simulink model "FOC_PI_5phase"  (R2024b)
settings: Solver=VariableStepAuto  StartTime=0.0  StopTime=0.5  RelTol=1e-3
InitFcn:
  | Pn=4;
  | Ld=1.35e-3;
  | Lq=1.35e-3;
  | R=2.875;
  | flux=0.05;
  | J=0.002;
  | B=0.02;
  | fc=470;
libraries: spsIGBTDiodeLib x10, slpidlib x3, simulink x1, spsDCVoltageSourceLib x1, spsPermanentMagnetSynchronousMachineLib x1, spsVoltageMeasurementLib x1, sps_lib x1
settings Model: Creator=23954  LastModifiedBy=23954

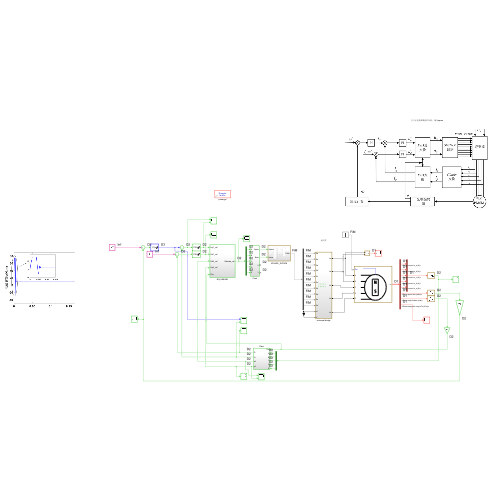
[thumbnail: Simulink's stored preview of the top-level diagram]
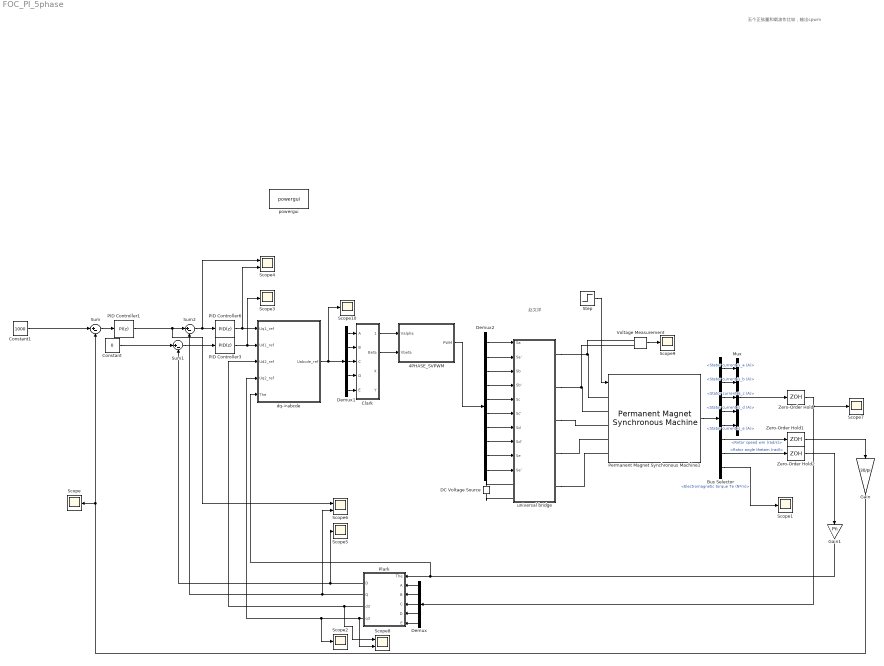
== system FOC_PI_5phase ==
  note: 赵文祥
  note: 五个正弦量和载波作比较，输出spwm
  4PHASE_SVPWM : Subsystem
  Bus Selector : BusSelector  OutputSignals=Stator current is_a (A),Stator current is_b (A),Stator current is_c (A),Stator current is_d (A),Stator current is_e (A),Rotor speed wm (rad/s),Rotor angle thetam (rad),Electromagnetic torque Te (N*m)
  Clark : Subsystem
  Constant : Constant  Value=0
  Constant1 : Constant  Value=1000
  DC Voltage Source : spsDCVoltageSourceLib/DC Voltage Source  Amplitude=311  Measurements=None
  Demux : Demux  Outputs=5
  Demux1 : Demux  Outputs=5
  Demux2 : Demux  Outputs=10
  Gain : Gain  Gain=30/pi
  Gain1 : Gain  Gain=Pn
  Mux : Mux  Inputs=5
  PID Controller1 : slpidlib/PID Controller  Controller=PI  Form=Parallel  TimeDomain=Discrete-time  UseExternalTs=off  SampleTime=1e-3  IntegratorMethod=Forward Euler  FilterMethod=Forward Euler  ControllerParametersSource=internal  P=5*J/1.5/Pn/flux  I=10*10*J/1.5/Pn/flux  UseKiTs=off  D=0  UseExternalDerivativeSource=off  N=100  UseFilter=on  TunerSelectOption=Transfer Function Based (PID Tuner App)  InitialConditionSource=internal  InitialConditionForIntegrator=0  InitialConditionForFilter=0  DifferentiatorICPrevScaledInput=0  ExternalReset=none  TrackingMode=off  Kt=1  LimitOutput=on  SatLimitsSource=internal  UpperSaturationLimit=150  LowerSaturationLimit=-150  LinearizeAsGain=on  AntiWindupMode=none  Kb=1  LimitIntegrator=off  UpperIntegratorSaturationLimit=inf  LowerIntegratorSaturationLimit=-inf  POutMin=[]  POutMax=[]  IOutMin=[]  IOutMax=[]  DOutMin=[]  DOutMax=[]  NOutMin=[]  NOutMax=[]  SumOutMin=[]  SumOutMax=[]  SaturationOutMin=[]  SaturationOutMax=[]  PParamMin=[]  PParamMax=[]  IParamMin=[]  IParamMax=[]  DParamMin=[]  DParamMax=[]  NParamMin=[]  NParamMax=[]  KbParamMin=[]  KbParamMax=[]  KtParamMin=[]  KtParamMax=[]  KbOutMin=[]  KbOutMax=[]  KtOutMin=[]  KtOutMax=[]  IntegratorOutMin=[]  IntegratorOutMax=[]  FilterOutMin=[]  FilterOutMax=[]  SumI1OutMin=[]  SumI1OutMax=[]  SumI2OutMin=[]  SumI2OutMax=[]  SumI3OutMin=[]  SumI3OutMax=[]  SumI4OutMin=[]  SumI4OutMax=[]  SumDOutMin=[]  SumDOutMax=[]  DifferentiatorOutMin=[]  DifferentiatorOutMax=[]  FilterDiffOutCoefMin=[]  FilterDiffOutCoefMax=[]  ReciprocalOutMin=[]  ReciprocalOutMax=[]  SumDenOutMin=[]  SumDenOutMax=[]  SumNumOutMin=[]  SumNumOutMax=[]  DivideOutMin=[]  DivideOutMax=[]  UdiffTsProdOutMin=[]  UdiffTsProdOutMax=[]  NTsProdOutMin=[]  NTsProdOutMax=[]  UintegralTsProdOutMin=[]  UintegralTsProdOutMax=[]  UngainTsProdOutMin=[]  UngainTsProdOutMax=[]  ClampingZeroOutDataTypeStr=Inherit: Inherit via back propagation  ClampingZeroOutMin=[]  ClampingZeroOutMax=[]  FilterDenConstantOutDataTypeStr=Inherit: Inherit via back propagation  FilterDenConstantOutMin=[]  FilterDenConstantOutMax=[]  PCopyOutDataTypeStr=Inherit: Inherit via back propagation  PCopyOutMin=[]  PCopyOutMax=[]  NCopyOutDataTypeStr=Inherit: Inherit via back propagation  NCopyOutMin=[]  NCopyOutMax=[]  IntegratorContinuousStateAttributes=''  IntegratorStateMustResolveToSignalObject=off  IntegratorRTWStateStorageClass=Auto  FilterContinuousStateAttributes=''  FilterStateMustResolveToSignalObject=off  FilterRTWStateStorageClass=Auto  ParallelPVariant=InternalParameters  IdealPVariant=Disabled  IVariant=InternalParameters  DVariant=Disabled  IntegratorVariant=Discrete  SatVariant=Enabled  AWVariant=Passthrough  PCopyVariant=Disabled  TRVariant=Disabled  FdbkBlocksVariant=Forward  IdealPFdbkVariant=Disabled  SatFdbkVariant=Disabled  DerivativeFilterVariant=Disabled  NVariant=Disabled  NCopyVariant=Disabled_SignalSpec  FilterICVariant=Disabled  IntegratorICVariant=InternalICs  ExternalResetVariant=Disabled  TRSumVariant=Passthrough  SumFdbkVariant=Disabled  SumVariant=Sum_PI  TsampFilterVariant=InternalTs  TsampNgainVariant=Passthrough  TsampIntegralVariant=Disabled_SignalSpec  ExternalSaturationOutDataTypeStr=Inherit: Same as second input  DerivativeSourceVariant=Disabled  PreIntVariant=InternalPreInt
  PID Controller3 : slpidlib/PID Controller  Controller=PID  Form=Parallel  TimeDomain=Discrete-time  UseExternalTs=off  SampleTime=1e-4  IntegratorMethod=Forward Euler  FilterMethod=Forward Euler  ControllerParametersSource=internal  P=2*pi*fc*Ld  I=2*pi*fc*R  UseKiTs=off  D=0  UseExternalDerivativeSource=off  N=100  UseFilter=on  TunerSelectOption=Transfer Function Based (PID Tuner App)  InitialConditionSource=internal  InitialConditionForIntegrator=0  InitialConditionForFilter=0  DifferentiatorICPrevScaledInput=0  ExternalReset=none  TrackingMode=off  Kt=1  LimitOutput=on  SatLimitsSource=internal  UpperSaturationLimit=150  LowerSaturationLimit=-150  LinearizeAsGain=on  AntiWindupMode=none  Kb=1  LimitIntegrator=off  UpperIntegratorSaturationLimit=inf  LowerIntegratorSaturationLimit=-inf  POutMin=[]  POutMax=[]  IOutMin=[]  IOutMax=[]  DOutMin=[]  DOutMax=[]  NOutMin=[]  NOutMax=[]  SumOutMin=[]  SumOutMax=[]  SaturationOutMin=[]  SaturationOutMax=[]  PParamMin=[]  PParamMax=[]  IParamMin=[]  IParamMax=[]  DParamMin=[]  DParamMax=[]  NParamMin=[]  NParamMax=[]  KbParamMin=[]  KbParamMax=[]  KtParamMin=[]  KtParamMax=[]  KbOutMin=[]  KbOutMax=[]  KtOutMin=[]  KtOutMax=[]  IntegratorOutMin=[]  IntegratorOutMax=[]  FilterOutMin=[]  FilterOutMax=[]  SumI1OutMin=[]  SumI1OutMax=[]  SumI2OutMin=[]  SumI2OutMax=[]  SumI3OutMin=[]  SumI3OutMax=[]  SumI4OutMin=[]  SumI4OutMax=[]  SumDOutMin=[]  SumDOutMax=[]  DifferentiatorOutMin=[]  DifferentiatorOutMax=[]  FilterDiffOutCoefMin=[]  FilterDiffOutCoefMax=[]  ReciprocalOutMin=[]  ReciprocalOutMax=[]  SumDenOutMin=[]  SumDenOutMax=[]  SumNumOutMin=[]  SumNumOutMax=[]  DivideOutMin=[]  DivideOutMax=[]  UdiffTsProdOutMin=[]  UdiffTsProdOutMax=[]  NTsProdOutMin=[]  NTsProdOutMax=[]  UintegralTsProdOutMin=[]  UintegralTsProdOutMax=[]  UngainTsProdOutMin=[]  UngainTsProdOutMax=[]  ClampingZeroOutDataTypeStr=Inherit: Inherit via back propagation  ClampingZeroOutMin=[]  ClampingZeroOutMax=[]  FilterDenConstantOutDataTypeStr=Inherit: Inherit via back propagation  FilterDenConstantOutMin=[]  FilterDenConstantOutMax=[]  PCopyOutDataTypeStr=Inherit: Inherit via back propagation  PCopyOutMin=[]  PCopyOutMax=[]  NCopyOutDataTypeStr=Inherit: Inherit via back propagation  NCopyOutMin=[]  NCopyOutMax=[]  IntegratorContinuousStateAttributes=''  IntegratorStateMustResolveToSignalObject=off  IntegratorRTWStateStorageClass=Auto  FilterContinuousStateAttributes=''  FilterStateMustResolveToSignalObject=off  FilterRTWStateStorageClass=Auto  ParallelPVariant=InternalParameters  IdealPVariant=Disabled  IVariant=InternalParameters  DVariant=InternalParameters  IntegratorVariant=Discrete  SatVariant=Enabled  AWVariant=Passthrough  PCopyVariant=Disabled  TRVariant=Disabled  FdbkBlocksVariant=Forward  IdealPFdbkVariant=Disabled  SatFdbkVariant=Disabled  DerivativeFilterVariant=ForwardEulerFilter  NVariant=InternalParameters  NCopyVariant=Disabled  FilterICVariant=InternalICsFilter  IntegratorICVariant=InternalICs  ExternalResetVariant=Disabled  TRSumVariant=Passthrough  SumFdbkVariant=Disabled  SumVariant=Sum_PID  TsampFilterVariant=InternalTs  TsampNgainVariant=Passthrough  TsampIntegralVariant=Disabled_SignalSpec  ExternalSaturationOutDataTypeStr=Inherit: Same as second input  DerivativeSourceVariant=ErrorSignal  PreIntVariant=InternalPreInt
  PID Controller6 : slpidlib/PID Controller  Controller=PID  Form=Parallel  TimeDomain=Discrete-time  UseExternalTs=off  SampleTime=1e-4  IntegratorMethod=Forward Euler  FilterMethod=Forward Euler  ControllerParametersSource=internal  P=2*pi*fc*Lq  I=2*pi*fc*R  UseKiTs=off  D=0  UseExternalDerivativeSource=off  N=100  UseFilter=on  TunerSelectOption=Transfer Function Based (PID Tuner App)  InitialConditionSource=internal  InitialConditionForIntegrator=0  InitialConditionForFilter=0  DifferentiatorICPrevScaledInput=0  ExternalReset=none  TrackingMode=off  Kt=1  LimitOutput=on  SatLimitsSource=internal  UpperSaturationLimit=150  LowerSaturationLimit=-150  LinearizeAsGain=on  AntiWindupMode=none  Kb=1  LimitIntegrator=off  UpperIntegratorSaturationLimit=inf  LowerIntegratorSaturationLimit=-inf  POutMin=[]  POutMax=[]  IOutMin=[]  IOutMax=[]  DOutMin=[]  DOutMax=[]  NOutMin=[]  NOutMax=[]  SumOutMin=[]  SumOutMax=[]  SaturationOutMin=[]  SaturationOutMax=[]  PParamMin=[]  PParamMax=[]  IParamMin=[]  IParamMax=[]  DParamMin=[]  DParamMax=[]  NParamMin=[]  NParamMax=[]  KbParamMin=[]  KbParamMax=[]  KtParamMin=[]  KtParamMax=[]  KbOutMin=[]  KbOutMax=[]  KtOutMin=[]  KtOutMax=[]  IntegratorOutMin=[]  IntegratorOutMax=[]  FilterOutMin=[]  FilterOutMax=[]  SumI1OutMin=[]  SumI1OutMax=[]  SumI2OutMin=[]  SumI2OutMax=[]  SumI3OutMin=[]  SumI3OutMax=[]  SumI4OutMin=[]  SumI4OutMax=[]  SumDOutMin=[]  SumDOutMax=[]  DifferentiatorOutMin=[]  DifferentiatorOutMax=[]  FilterDiffOutCoefMin=[]  FilterDiffOutCoefMax=[]  ReciprocalOutMin=[]  ReciprocalOutMax=[]  SumDenOutMin=[]  SumDenOutMax=[]  SumNumOutMin=[]  SumNumOutMax=[]  DivideOutMin=[]  DivideOutMax=[]  UdiffTsProdOutMin=[]  UdiffTsProdOutMax=[]  NTsProdOutMin=[]  NTsProdOutMax=[]  UintegralTsProdOutMin=[]  UintegralTsProdOutMax=[]  UngainTsProdOutMin=[]  UngainTsProdOutMax=[]  ClampingZeroOutDataTypeStr=Inherit: Inherit via back propagation  ClampingZeroOutMin=[]  ClampingZeroOutMax=[]  FilterDenConstantOutDataTypeStr=Inherit: Inherit via back propagation  FilterDenConstantOutMin=[]  FilterDenConstantOutMax=[]  PCopyOutDataTypeStr=Inherit: Inherit via back propagation  PCopyOutMin=[]  PCopyOutMax=[]  NCopyOutDataTypeStr=Inherit: Inherit via back propagation  NCopyOutMin=[]  NCopyOutMax=[]  IntegratorContinuousStateAttributes=''  IntegratorStateMustResolveToSignalObject=off  IntegratorRTWStateStorageClass=Auto  FilterContinuousStateAttributes=''  FilterStateMustResolveToSignalObject=off  FilterRTWStateStorageClass=Auto  ParallelPVariant=InternalParameters  IdealPVariant=Disabled  IVariant=InternalParameters  DVariant=InternalParameters  IntegratorVariant=Discrete  SatVariant=Enabled  AWVariant=Passthrough  PCopyVariant=Disabled  TRVariant=Disabled  FdbkBlocksVariant=Forward  IdealPFdbkVariant=Disabled  SatFdbkVariant=Disabled  DerivativeFilterVariant=ForwardEulerFilter  NVariant=InternalParameters  NCopyVariant=Disabled  FilterICVariant=InternalICsFilter  IntegratorICVariant=InternalICs  ExternalResetVariant=Disabled  TRSumVariant=Passthrough  SumFdbkVariant=Disabled  SumVariant=Sum_PID  TsampFilterVariant=InternalTs  TsampNgainVariant=Passthrough  TsampIntegralVariant=Disabled_SignalSpec  ExternalSaturationOutDataTypeStr=Inherit: Same as second input  DerivativeSourceVariant=ErrorSignal  PreIntVariant=InternalPreInt
  Permanent Magnet Synchronous Machine1 : spsPermanentMagnetSynchronousMachineLib/Permanent Magnet Synchronous Machine  NbPhases=5  FluxDistribution=Sinusoidal  RotorType=Round  MechanicalLoad=Torque Tm  PresetModel=No  ShowDetailedParameters=on  MeasurementBus=off  Resistance=2.875  Inductance=8.5e-3  dqInductances=[8.5e-3,8.5e-3]  La=1.35e-3  MachineConstant=Flux linkage established by magnets (V.s)  Flux=0.05  VoltageCst=24.6211  TorqueCst=0.5  Flat=120  Mechanical=[0.002 0.02 4 0]  PolePairs=4  InitialConditions=[0,0, 0,0]  InitialConditions5ph=[0 0 0 0 0 0]  RefAngle=Aligned with phase A axis (original Park)  IterativeDiscreteModel=Trapezoidal non iterative  TsBlock=-1  TsPowergui=0
  Plark : Subsystem
  Scope{,1..3,5,7,9..10} (8 alike) : Scope
  Scope4 : Scope  NumInputPorts=2
  Scope6 : Scope  NumInputPorts=2
  Scope8 : Scope  NumInputPorts=2
  Step : Step  Time=0.2  After=5  SampleTime=0
  Sum : Sum  Inputs=|+-
  Sum1 : Sum  Inputs=|+-
  Sum2 : Sum  Inputs=|+-
  Voltage Measurement : spsVoltageMeasurementLib/Voltage Measurement  PhasorSimulation=off  OutputType=Complex  PSBequivalent=0
  Zero-Order Hold : ZeroOrderHold  SampleTime=1e-4
  Zero-Order Hold1 : ZeroOrderHold  SampleTime=1e-4
  Zero-Order Hold2 : ZeroOrderHold  SampleTime=1e-4
  dq->abcde : Subsystem
  powergui : sps_lib/powergui  Priority=1  SimulationMode=Discrete  SampleTime=1e-6  frequency=60  Iterations=50  frequencyindice=0  Pbase=100e6  ErrMax=1e-4  UnitsV=kV  UnitsW=MW  buscounter=0  FunctionMessages=off  echomessages=off  EnableUseOfTLC=off  CurrentSourceSwitches=off  DisableSnubberDevices=off  DisableRonSwitches=off  DisableVfSwitches=off  DisplayEquations=off  AutomaticDiscreteSolvers=off  SolverType=Tustin/Backward Euler (TBE)  Interpol=off  ExternalGateDelay=off  methode=off  Ts=100  x0status=blocks  SPID=on  SwTol=0  HookPort=off  NonlinearTolerance=1e-4  nMaxIteration=100  ContinueOnMaxIteration=off  RestoreLinks=warning  ResistiveCurrentMeasurement=off  Frange=[0:2:500]  Ylog=off  Xlog=on  ShowGrid=off  save=off  variable=ZData  structure=0  ZoomFFT=off  StartTime=0.0  cycles=1  DisplayStyle=1  fundamental=60  FreqAxis=off  MaxFrequency=1000  frequencyindicesteady=1  RmsSteady=1  display=off
  universal bridge : Subsystem
  wires:
  Gain/1 -> Sum/2, Scope/1
  Bus Selector/4 -> Mux/4  "<Stator current is_d (A)>"
  PID Controller1/1 -> Scope6/1, Sum2/1
  Bus Selector/2 -> Mux/2  "<Stator current is_b (A)>"
  Zero-Order Hold2/1 -> Gain1/1
  Bus Selector/5 -> Mux/5  "<Stator current is_e (A)>"
  Permanent Magnet Synchronous Machine1/1 -> Bus Selector/1
  Bus Selector/6 -> Zero-Order Hold1/1  "<Rotor speed wm (rad/s)>"
  Sum/1 -> PID Controller1/1
  Bus Selector/7 -> Zero-Order Hold2/1  "<Rotor angle thetam (rad)>"
  Bus Selector/1 -> Mux/1  "<Stator current is_a (A)>"
  Mux/1 -> Zero-Order Hold/1
  Zero-Order Hold1/1 -> Gain/1
  Zero-Order Hold/1 -> Scope7/1, Demux/1
  Bus Selector/3 -> Mux/3  "<Stator current is_c (A)>"
  Constant1/1 -> Sum/1
  Constant/1 -> Sum1/1
  Gain1/1 -> dq->abcde/5(The), Plark/1(The)
  Demux/5 -> Plark/6(E)
  Demux/4 -> Plark/5(D)
  Demux/3 -> Plark/4(C)
  Demux/2 -> Plark/3(B)
  Demux/1 -> Plark/2(A)
  Plark/2(Q) -> Scope6/2, Sum2/2
  Plark/1("D ") -> Scope5/1, Sum1/2
  Plark/3(d3) -> dq->abcde/3(Ud2_ref), Scope8/1
  Plark/4(q3) -> Scope8/2, dq->abcde/4(Uq2_ref), Scope2/1
  dq->abcde/1(Uabcde_ref) -> Scope10/1, Demux1/1
  Demux1/5 -> Clark/5(E)
  Demux1/4 -> Clark/4(D)
  Demux1/3 -> Clark/3(C)
  Demux1/2 -> Clark/2(B)
  Demux1/1 -> Clark/1(A)
  Sum1/1 -> PID Controller3/1
  Clark/1(Alpha) -> 4PHASE_SVPWM/1(Valpha)
  Clark/2(Beta) -> 4PHASE_SVPWM/2(Vbeta)
  4PHASE_SVPWM/1(PWM) -> Demux2/1
  Demux2/1 -> universal bridge/1(Sa)
  Demux2/2 -> universal bridge/2(Sa')
  Demux2/3 -> universal bridge/3(Sb)
  Demux2/4 -> universal bridge/4(Sb')
  Demux2/5 -> universal bridge/5(Sc)
  Demux2/6 -> universal bridge/6(Sc')
  Demux2/7 -> universal bridge/7(Sd)
  Demux2/8 -> universal bridge/8(Sd')
  Demux2/9 -> universal bridge/9(Se)
  Demux2/10 -> universal bridge/10(Se')
  PID Controller3/1 -> Scope3/1, dq->abcde/2(Ud1_ref)
  Bus Selector/8 -> Scope1/1  "<Electromagnetic torque Te (N*m)>"
  Step/1 -> Permanent Magnet Synchronous Machine1/1
  Sum2/1 -> Scope4/1, PID Controller6/1
  PID Controller6/1 -> Scope4/2, dq->abcde/1("Uq1_ref ")
  Voltage Measurement/1 -> Scope9/1
  connections:
  universal bridge/RConn5 -- Permanent Magnet Synchronous Machine1/LConn5
  universal bridge/RConn2 -- Voltage Measurement/LConn2 -- Permanent Magnet Synchronous Machine1/LConn2
  universal bridge/RConn3 -- Permanent Magnet Synchronous Machine1/LConn3
  universal bridge/RConn1 -- Voltage Measurement/LConn1 -- Permanent Magnet Synchronous Machine1/LConn1
  universal bridge/RConn4 -- Permanent Magnet Synchronous Machine1/LConn4
  DC Voltage Source/RConn1 -- universal bridge/LConn1
  DC Voltage Source/LConn1 -- universal bridge/LConn2

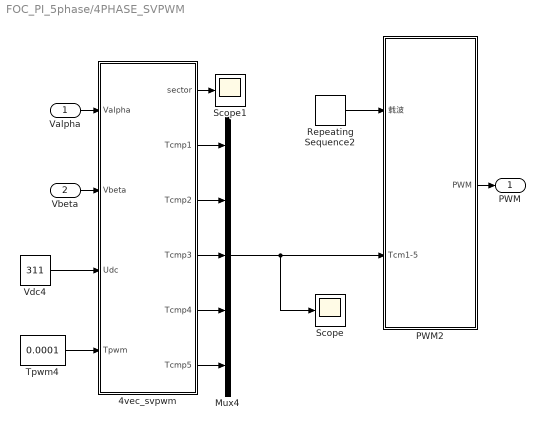
== system FOC_PI_5phase/4PHASE_SVPWM ==
  Valpha : Inport
  Vbeta : Inport  Port=2
  4vec_svpwm : MATLAB Function  TreatAsAtomicUnit=on
  Mux4 : Mux  Inputs=5
  PWM2 : Subsystem
  Repeating Sequence2 : simulink/Sources/Repeating Sequence  rep_seq_t=[0 5/100000 1/10000]  rep_seq_y=[0 5/100000 0]
  Scope : Scope
  Scope1 : Scope
  Tpwm4 : Constant  Value=0.0001
  Vdc4 : Constant  Value=311
  PWM : Outport
  wires:
  Tpwm4/1 -> 4vec_svpwm/4(Tpwm)
  4vec_svpwm/5(Tcmp4) -> Mux4/4
  4vec_svpwm/6(Tcmp5) -> Mux4/5
  4vec_svpwm/2(Tcmp1) -> Mux4/1
  Vdc4/1 -> 4vec_svpwm/3(Udc)
  Repeating Sequence2/1 -> PWM2/1(载波)
  4vec_svpwm/3(Tcmp2) -> Mux4/2
  Mux4/1 -> Scope/1, PWM2/2(Tcm1-5)
  4vec_svpwm/4(Tcmp3) -> Mux4/3
  4vec_svpwm/1(sector) -> Scope1/1
  Vbeta/1 -> 4vec_svpwm/2(Vbeta)
  PWM2/1(PWM) -> PWM/1
  Valpha/1 -> 4vec_svpwm/1(Valpha)

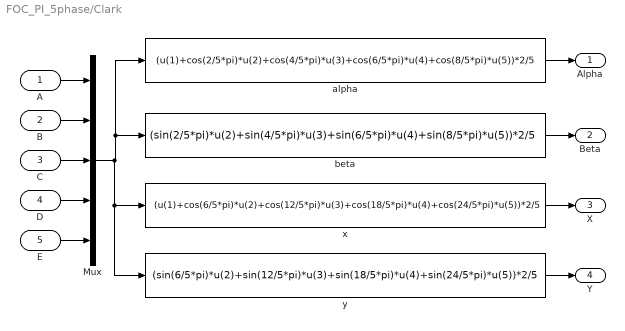
== system FOC_PI_5phase/Clark ==
  A : Inport
  B : Inport  Port=2
  C : Inport  Port=3
  D : Inport  Port=4
  E : Inport  Port=5
  Mux : Mux  Inputs=5
  alpha : Fcn  Expr=(u(1)+cos(2/5*pi)*u(2)+cos(4/5*pi)*u(3)+cos(6/5*pi)*u(4)+cos(8/5*pi)*u(5))*2/5
  beta : Fcn  Expr=(sin(2/5*pi)*u(2)+sin(4/5*pi)*u(3)+sin(6/5*pi)*u(4)+sin(8/5*pi)*u(5))*2/5
  "x " : Fcn  Expr=(u(1)+cos(6/5*pi)*u(2)+cos(12/5*pi)*u(3)+cos(18/5*pi)*u(4)+cos(24/5*pi)*u(5))*2/5
  "y " : Fcn  Expr=(sin(6/5*pi)*u(2)+sin(12/5*pi)*u(3)+sin(18/5*pi)*u(4)+sin(24/5*pi)*u(5))*2/5
  Alpha : Outport
  Beta : Outport  Port=2
  X : Outport  Port=3
  Y : Outport  Port=4
  wires:
  "y "/1 -> Y/1
  "x "/1 -> X/1
  Mux/1 -> beta/1, alpha/1, "y "/1, "x "/1
  E/1 -> Mux/5
  D/1 -> Mux/4
  beta/1 -> Beta/1
  A/1 -> Mux/1
  C/1 -> Mux/3
  B/1 -> Mux/2
  alpha/1 -> Alpha/1

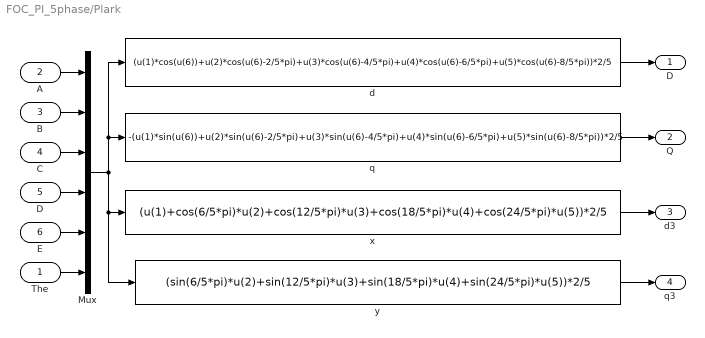
== system FOC_PI_5phase/Plark ==
  The : Inport
  A : Inport  Port=2
  B : Inport  Port=3
  C : Inport  Port=4
  D : Inport  Port=5
  E : Inport  Port=6
  Mux : Mux  Inputs=6
  d : Fcn  Expr=(u(1)*cos(u(6))+u(2)*cos(u(6)-2/5*pi)+u(3)*cos(u(6)-4/5*pi)+u(4)*cos(u(6)-6/5*pi)+u(5)*cos(u(6)-8/5*pi))*2/5
  q : Fcn  Expr=-(u(1)*sin(u(6))+u(2)*sin(u(6)-2/5*pi)+u(3)*sin(u(6)-4/5*pi)+u(4)*sin(u(6)-6/5*pi)+u(5)*sin(u(6)-8/5*pi))*2/5
  "x " : Fcn  Expr=(u(1)+cos(6/5*pi)*u(2)+cos(12/5*pi)*u(3)+cos(18/5*pi)*u(4)+cos(24/5*pi)*u(5))*2/5
  "y " : Fcn  Expr=(sin(6/5*pi)*u(2)+sin(12/5*pi)*u(3)+sin(18/5*pi)*u(4)+sin(24/5*pi)*u(5))*2/5
  "D " : Outport
  Q : Outport  Port=2
  d3 : Outport  Port=3
  q3 : Outport  Port=4
  wires:
  "y "/1 -> q3/1
  "x "/1 -> d3/1
  q/1 -> Q/1
  Mux/1 -> "x "/1, "y "/1, d/1, q/1
  The/1 -> Mux/6
  E/1 -> Mux/5
  D/1 -> Mux/4
  A/1 -> Mux/1
  C/1 -> Mux/3
  B/1 -> Mux/2
  d/1 -> "D "/1

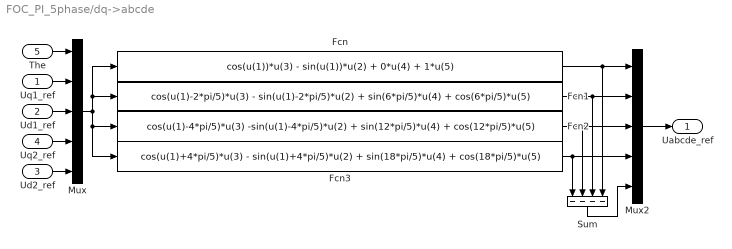
== system FOC_PI_5phase/dq->abcde ==
  "Uq1_ref " : Inport
  Ud1_ref : Inport  Port=2
  Ud2_ref : Inport  Port=3
  Uq2_ref : Inport  Port=4
  The : Inport  Port=5
  Fcn : Fcn  Expr=cos(u(1))*u(3) - sin(u(1))*u(2) + 0*u(4) + 1*u(5)
  Fcn1 : Fcn  Expr=cos(u(1)-2*pi/5)*u(3) - sin(u(1)-2*pi/5)*u(2) + sin(6*pi/5)*u(4) + cos(6*pi/5)*u(5)
  Fcn2 : Fcn  Expr=cos(u(1)-4*pi/5)*u(3) -sin(u(1)-4*pi/5)*u(2) + sin(12*pi/5)*u(4) + cos(12*pi/5)*u(5)
  Fcn3 : Fcn  Expr=cos(u(1)+4*pi/5)*u(3) - sin(u(1)+4*pi/5)*u(2) + sin(18*pi/5)*u(4) + cos(18*pi/5)*u(5)
  Mux : Mux  Inputs=5
  Mux2 : Mux  Inputs=5
  Sum : Sum  Inputs=----  InputSameDT=on  SaturateOnIntegerOverflow=on  OutDataTypeStr=Inherit: Same as first input
  Uabcde_ref : Outport  InitialOutput=0
  wires:
  Sum/1 -> Mux2/5
  Fcn1/1 -> Mux2/2, Sum/3
  Fcn2/1 -> Mux2/3, Sum/2
  Fcn3/1 -> Mux2/4, Sum/1
  Mux/1 -> Fcn2/1, Fcn3/1, Fcn/1, Fcn1/1
  Fcn/1 -> Sum/4, Mux2/1
  The/1 -> Mux/1
  "Uq1_ref "/1 -> Mux/2
  Ud1_ref/1 -> Mux/3
  Uq2_ref/1 -> Mux/4
  Ud2_ref/1 -> Mux/5
  Mux2/1 -> Uabcde_ref/1

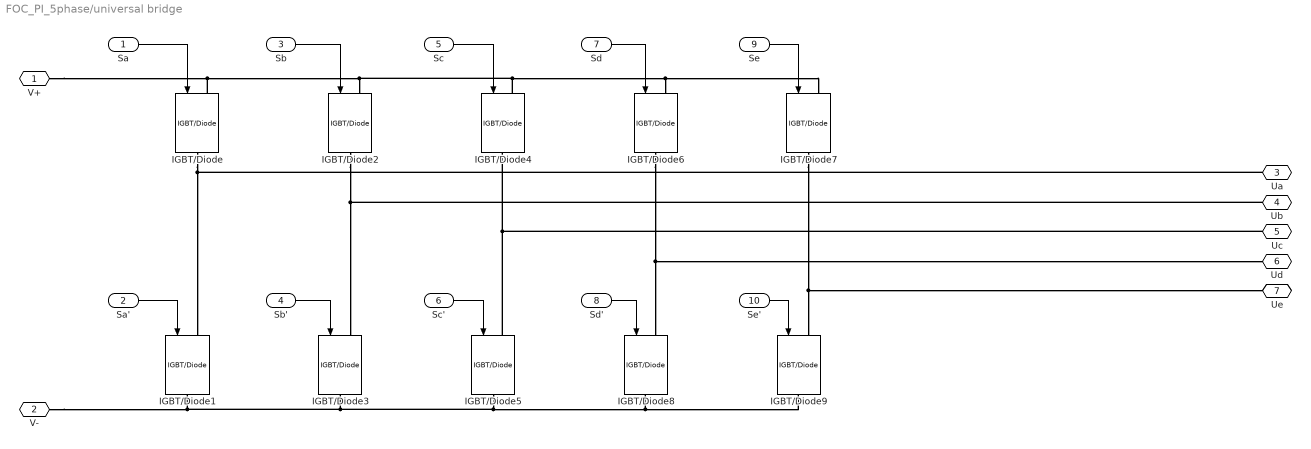
== system FOC_PI_5phase/universal bridge ==
  Sa : Inport
  Sa' : Inport  Port=2
  Sb : Inport  Port=3
  Sb' : Inport  Port=4
  Sc : Inport  Port=5
  Sc' : Inport  Port=6
  Sd : Inport  Port=7
  Sd' : Inport  Port=8
  Se : Inport  Port=9
  Se' : Inport  Port=10
  IGBT/Diode{,1..9} (10 alike) : spsIGBTDiodeLib/IGBT//Diode  Ron=1e-3  Rs=1e5  Cs=inf  Measurements=off
  V+ : PMIOPort  Side=Left
  V- : PMIOPort  Port=2  Side=Left
  Ua : PMIOPort  Port=3  Side=Right
  Ub : PMIOPort  Port=4  Side=Right
  Uc : PMIOPort  Port=5  Side=Right
  Ud : PMIOPort  Port=6  Side=Right
  Ue : PMIOPort  Port=7  Side=Right
  wires:
  Sa/1 -> IGBT/Diode/1
  Sb/1 -> IGBT/Diode2/1
  Sb'/1 -> IGBT/Diode3/1
  Sa'/1 -> IGBT/Diode1/1
  Sc'/1 -> IGBT/Diode5/1
  Sc/1 -> IGBT/Diode4/1
  Sd/1 -> IGBT/Diode6/1
  Se/1 -> IGBT/Diode7/1
  Sd'/1 -> IGBT/Diode8/1
  Se'/1 -> IGBT/Diode9/1
  connections:
  IGBT/Diode2/RConn1 -- Ub/RConn1 -- IGBT/Diode3/LConn1
  IGBT/Diode2/LConn1 -- IGBT/Diode7/LConn1 -- IGBT/Diode6/LConn1 -- IGBT/Diode4/LConn1 -- V+/RConn1 -- IGBT/Diode/LConn1
  IGBT/Diode5/RConn1 -- IGBT/Diode9/RConn1 -- IGBT/Diode8/RConn1 -- IGBT/Diode3/RConn1 -- V-/RConn1 -- IGBT/Diode1/RConn1
  IGBT/Diode5/LConn1 -- IGBT/Diode4/RConn1 -- Uc/RConn1
  IGBT/Diode/RConn1 -- IGBT/Diode1/LConn1 -- Ua/RConn1
  IGBT/Diode6/RConn1 -- IGBT/Diode8/LConn1 -- Ud/RConn1
  IGBT/Diode7/RConn1 -- Ue/RConn1 -- IGBT/Diode9/LConn1

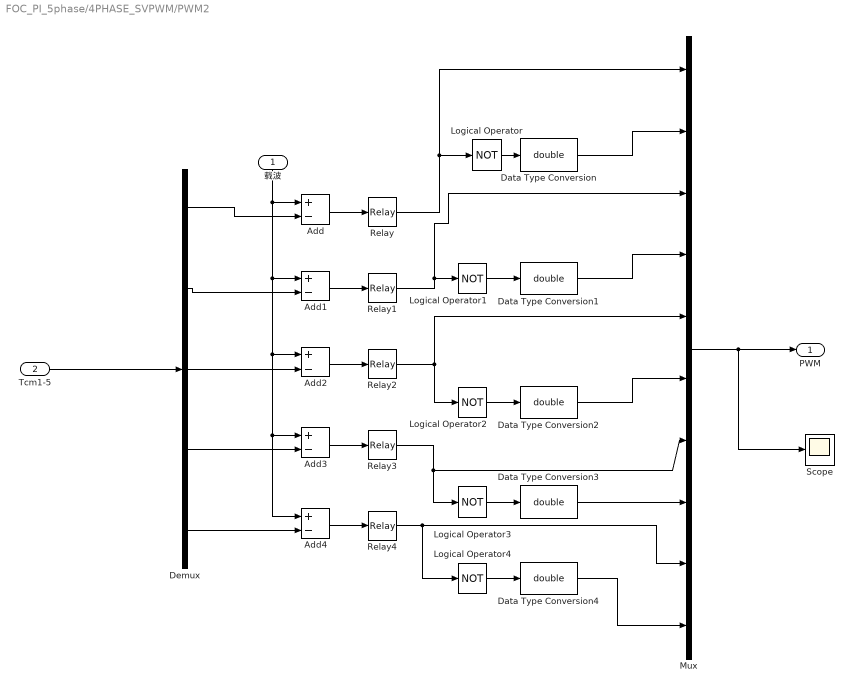
== system FOC_PI_5phase/4PHASE_SVPWM/PWM2 ==
  载波 : Inport
  Tcm1-5 : Inport  Port=2
  Add{,1..4} (5 alike) : Sum  Inputs=+-
  Data Type Conversion{,1..4} (5 alike) : DataTypeConversion  OutDataTypeStr=double  SaturateOnIntegerOverflow=off  RndMeth=Floor
  Demux : Demux  Outputs=5
  Logical Operator{,1..4} (5 alike) : Logic  Operator=NOT  AllPortsSameDT=off  OutDataTypeStr=boolean
  Mux : Mux  Inputs=10
  Relay{,1..4} (5 alike) : Relay  OffSwitchValue=-eps
  Scope : Scope
  PWM : Outport
  wires:
  Data Type Conversion4/1 -> Mux/10
  Relay4/1 -> Logical Operator4/1, Mux/9
  Logical Operator4/1 -> Data Type Conversion4/1
  Data Type Conversion3/1 -> Mux/8
  Relay3/1 -> Logical Operator3/1, Mux/7
  Logical Operator3/1 -> Data Type Conversion3/1
  Add4/1 -> Relay4/1
  Add3/1 -> Relay3/1
  Demux/4 -> Add3/2
  Demux/5 -> Add4/2
  Tcm1-5/1 -> Demux/1
  载波/1 -> Add1/1, Add2/1, Add3/1, Add4/1, Add/1
  Add/1 -> Relay/1
  Add2/1 -> Relay2/1
  Add1/1 -> Relay1/1
  Logical Operator/1 -> Data Type Conversion/1
  Logical Operator1/1 -> Data Type Conversion1/1
  Logical Operator2/1 -> Data Type Conversion2/1
  Data Type Conversion2/1 -> Mux/6
  Data Type Conversion1/1 -> Mux/4
  Data Type Conversion/1 -> Mux/2
  Mux/1 -> Scope/1, PWM/1
  Relay/1 -> Logical Operator/1, Mux/1
  Relay1/1 -> Logical Operator1/1, Mux/3
  Relay2/1 -> Logical Operator2/1, Mux/5
  Demux/1 -> Add/2
  Demux/2 -> Add1/2
  Demux/3 -> Add2/2

== matlab function FOC_PI_5phase/4PHASE_SVPWM/4vec_svpwm ==
  data: Valpha input; sector output; Vbeta input; Udc input; Tpwm input; Tcmp1 output; Tcmp2 output; Tcmp3 output; Tcmp4 output; Tcmp5 output
function [sector,Tcmp1,Tcmp2,Tcmp3,Tcmp4,Tcmp5]  = fcn(Valpha,Vbeta,Udc,Tpwm)

sector = 0;
P = 0;
Tcmp1 = 0;
Tcmp2 = 0;
Tcmp3 = 0;
Tcmp4 = 0;
Tcmp5 = 0;
T1=0;
T2=0;
T3=0;
T4=0;
T5=0;


%========Parameters statement================
%参考电压
Vref1 = Vbeta;
Vref2 = -Valpha*sin(2*pi/10)+Vbeta*cos(2*pi/5);
Vref3 = -Valpha*sin(4*pi/5)-Vbeta*cos(pi/5);
Vref4 = Valpha*sin(pi/5)-Vbeta*cos(pi/5);
Vref5 = Valpha*sin(2*pi/5)+Vbeta*cos(2*pi/5);

%========sign function=================
%扇区判断
if (Vref1>0)
    Q = 1;
else
    Q = 0;
end

if (Vref2>0)
    W = 1;
else
    W = 0;
end

if (Vref3>0)
    Y = 1;
else
    Y = 0;
end

if (Vref4>0)
    R = 1;
else
    R = 0;
end

if (Vref5>0)
    T = 1;
else
    T = 0;
end

sector = Q+2*W+4*Y+6*R+8*T;
switch(sector)
    case 15
        sector=1;
    case 9
        sector=2;
    case 11
        sector=3;
    case 3
        sector=4;
    case 7
        sector=5;
    case 6
        sector=6;
    case 12
        sector=7;
    case 10
        sector=8;
    case 18
        sector=9;
    otherwise
        sector=10;
end


%======== A B C D E calculation=============
%3.3各矢量作用时间计算（7）

A = Vbeta*1.902*Tpwm/Udc;
B = (Valpha*sin(pi/5)-Vbeta*cos(pi/5))*1.902*Tpwm/Udc;
C = (Valpha*cos(pi/10)-Vbeta*sin(pi/10))*1.902*Tpwm/Udc;
D = (Valpha*cos(pi/10)+Vbeta*sin(pi/10))*1.902*Tpwm/Udc;
E = (Valpha*sin(pi/5)+Vbeta*cos(pi/5))*1.902*Tpwm/Udc;

%==========Duty ratio calculation================
%根据sector查表（2）
switch (sector)
    case 1
        T1 = A; T2 = B; T3 = 0.618*B;T4 = 0.618*A;
    case 2
        T1 = C; T2 = -B; T3 = -0.618*B;T4 = 0.618*C;
    case 3
        T1 = -C; T2 = D;  T3 = 0.618*D;T4 = -0.618*C;
    case 4
        T1 = E; T2 = -D; T3 = -0.618*D;T4 = 0.618*E;
    case 5
        T1 = -E; T2 = A; T3 = 0.618*A;T4 = -0.618*E;
    case 6
        T1 = -B; T2 = -A; T3 = -0.618*A;T4 = -0.618*B;
    case 7
        T1 = B; T2 = -C; T3 = -0.618*C;T4 = 0.618*B;
    case 8
        T1 =-D; T2 =C; T3 = 0.618*C;T4 = -0.618*D;
    case 9
        T1 = D; T2 = -E; T3 = -0.618*E;T4 = 0.618*D;
    case 10
        T1 = -A; T2 = E; T3 = 0.618*E;T4 = -0.618*A;
end
%过调制处理(8-16)
if T1+T2+T3+T4>Tpwm
    T1=T1*Tpwm/(T1+T2+T3+T4);
    T2=T2*Tpwm/(T1+T2+T3+T4);
    T3=T3*Tpwm/(T1+T2+T3+T4);
    T4=T4*Tpwm/(T1+T2+T3+T4);
else
    T1=T1;
    T2=T2;
    T3=T3;
    T4=T4;
end
%ta为Tacom，式（8）
ta = (Tpwm-(T1+T2+T3+T4))/4.0;
tb = ta+T3/2;
tc = tb+T1/2;
td = tc+T2/2;
te = td+T4/2;
%==========Duty ratio calculation================
%各扇区时间切换点，表（3）
switch (sector)
    case 1
        Tcmp1=ta;
        Tcmp2=tb;
        Tcmp3=td;
        Tcmp4=te;
        Tcmp5=tc;

    case 2
        Tcmp1=tb;
        Tcmp2=ta;
        Tcmp3=tc;
        Tcmp4=te;
        Tcmp5=td;

    case 3
        Tcmp1=tc;
        Tcmp2=ta;
        Tcmp3=tb;
        Tcmp4=td;
        Tcmp5=te;

    case 4
        Tcmp1=td;
        Tcmp2=tb;
        Tcmp3=ta;
        Tcmp4=tc;
        Tcmp5=te;

    case 5
        Tcmp1=te;
        Tcmp2=tc;
        Tcmp3=ta;
        Tcmp4=tb;
        Tcmp5=td;

    case 6
        Tcmp1=te;
        Tcmp2=td;
        Tcmp3=tb;
        Tcmp4=ta;
        Tcmp5=tc;

    case 7
        Tcmp1=td;
        Tcmp2=te;
        Tcmp3=tc;
        Tcmp4=ta;
        Tcmp5=tb;

    case 8
        Tcmp1=tc;
        Tcmp2=te;
        Tcmp3=td;
        Tcmp4=tb;
        Tcmp5=ta;

    case 9
        Tcmp1=tb;
        Tcmp2=td;
        Tcmp3=te;
        Tcmp4=tc;
        Tcmp5=ta;

    case 10
        Tcmp1=ta;
        Tcmp2=tc;
        Tcmp3=te;
        Tcmp4=td;
        Tcmp5=tb;
end
